simulink model "tp3_schema"  (R2018b)
settings: Solver=VariableStepAuto  StartTime=0.0  StopTime=10  MaxStep=0.01  RelTol=1e-3
values from neighbouring files (symbols this model uses):
  k1 = 56.25/(10*pi)    (= 1.79049310978)    [parametres_tp3.m]
  k2 = 1/2    (= 0.5)    [parametres_tp3.m]
settings Model: Creator=e12108993  LastModifiedBy=e12108993

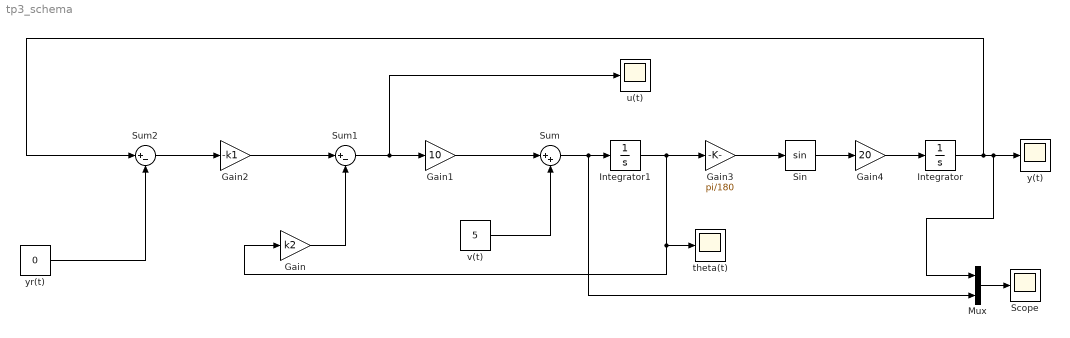
== system tp3_schema ==
  Gain : Gain  Gain=k2
  Gain1 : Gain  Gain=10
  Gain2 : Gain  Gain=-k1
  Gain3 : Gain  Gain=pi/180
  Gain4 : Gain  Gain=20
  Integrator : Integrator
  Integrator1 : Integrator
  Mux : Mux  Inputs=2
  Scope : Scope
  Sin : Trigonometry
  Sum : Sum  Inputs=|++
  Sum1 : Sum  Inputs=|+-
  Sum2 : Sum  Inputs=|+-
  theta(t) : Scope
  "u(t) " : Scope
  v(t) : Constant  Value=5
  "y(t) " : Scope
  "yr(t) " : Constant  Value=0
  wires:
  "yr(t) "/1 -> Sum2/2
  Sum2/1 -> Gain2/1
  Gain2/1 -> Sum1/1
  v(t)/1 -> Sum/2
  Gain/1 -> Sum1/2
  Sum1/1 -> "u(t) "/1, Gain1/1
  Gain1/1 -> Sum/1
  Sum/1 -> Mux/2, Integrator1/1
  Integrator1/1 -> theta(t)/1, Gain/1, Gain3/1
  Gain3/1 -> Sin/1
  Sin/1 -> Gain4/1
  Gain4/1 -> Integrator/1
  Integrator/1 -> Sum2/1, Mux/1, "y(t) "/1
  Mux/1 -> Scope/1
